simulink model "Three_point_guidance_law"  (R2024b)
settings: Solver=FixedStepAuto  StartTime=0.0  StopTime=200  FixedStep=0.01  RelTol=1e-3
settings Model: Creator=Acer  LastModifiedBy=Acer
settings DataIOCC: ReturnWorkspaceOutputs=off

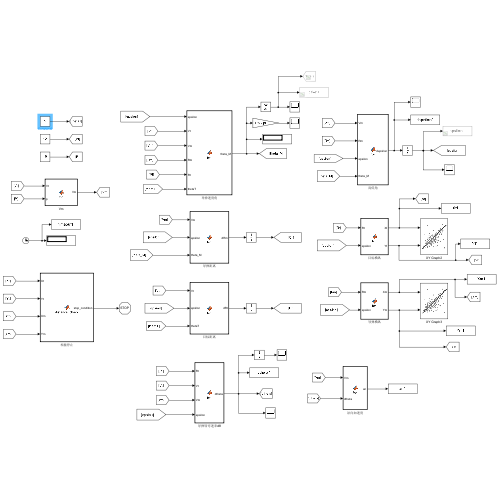
[thumbnail: Simulink's stored preview of the top-level diagram]
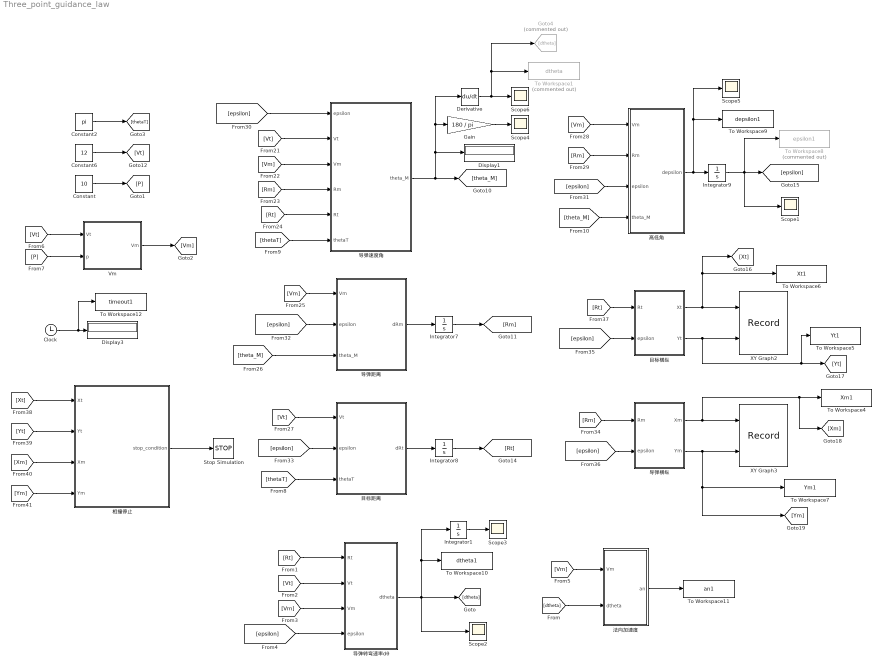
== system Three_point_guidance_law ==
  Clock : Clock
  Constant : Constant  Value=10
  Constant2 : Constant  Value=pi
  Constant6 : Constant  Value=12
  Derivative : Derivative
  Display1 : Display
  Display3 : Display
  Gain : Gain  Gain=180 / pi
  Goto4 : Goto  Commented=on  GotoTag=dtheta
  Integrator1 : Integrator  InitialCondition=70 * pi / 180
  Integrator7 : Integrator  InitialCondition=50
  Integrator8 : Integrator  InitialCondition=3000
  Integrator9 : Integrator  InitialCondition=70 * pi / 180
  Scope{1..6} (6 alike) : Scope
  Stop Simulation : Stop
  To Workspace1 : ToWorkspace  Commented=on  VariableName=dtheta  SaveFormat=Timeseries  SampleTime=-1
  To Workspace10 : ToWorkspace  VariableName=dtheta1  SaveFormat=Timeseries  SampleTime=-1
  To Workspace11 : ToWorkspace  VariableName=an1  SaveFormat=Timeseries  SampleTime=-1
  To Workspace12 : ToWorkspace  VariableName=timeout1  SaveFormat=Timeseries  SampleTime=-1
  To Workspace4 : ToWorkspace  VariableName=Xm1  SaveFormat=Timeseries  SampleTime=-1
  To Workspace5 : ToWorkspace  VariableName=Yt1  SaveFormat=Timeseries  SampleTime=-1
  To Workspace6 : ToWorkspace  VariableName=Xt1  SaveFormat=Timeseries  SampleTime=-1
  To Workspace7 : ToWorkspace  VariableName=Ym1  SaveFormat=Timeseries  SampleTime=-1
  To Workspace8 : ToWorkspace  Commented=on  VariableName=epsilon1  SaveFormat=Timeseries  SampleTime=-1
  To Workspace9 : ToWorkspace  VariableName=depsilon1  SaveFormat=Timeseries  SampleTime=-1
  Vm : MATLAB Function  TreatAsAtomicUnit=on
  XY Graph2 : Record  FileSettingsInternal="{\"entries\":[{\"content\":{\"excelSettings\":{\"content\":{},\"type\":\"Streamout.ExcelSettings\"}},\"type\":\"Streamout.FileSettingStorage\",\"uuid\":\"\"}],\"packageUris\":[\"http:\\/\\/schema.mathworks.com\\/mf0\\/streamout_blocks\\/R2020a\"],\"version\":\"1.0\"}"  Layout=[1 1]  SignalsInternal="{\"entries\":[{\"content\":{\"signals\":[{\"content\":{\"blockPath\":[],\"dimensions\":[1],\"domain\":\"\",\"lineColor\":\"#a2142f\",\"plots\":[ 1 ],\"port\":1,\"signalID\":1,\"signalName\":\"目标横纵:1\"},\"type\":\"RecordBlkView.Signal\",\"uuid\":\"\"},{\"content\":{\"blockPath\":[],\"dimensions\":[1],\"domain\":\"\",\"lineColor\":\"#139fff\",\"plots\":[ 1 ],\"port\":2,\"signalID\":2,\"signalName\":\"目标横纵:2\"},\"type\":\"RecordBlkView.Signal\",\"uuid\":\"\"}]},\"type\":\"RecordBlkView.InputSignals\",\"uuid\":\"\"}],\"packageUris\":[\"http:\\/\\/schema.mathworks.com\\/mf0\\/streamout_blocks\\/R2020a\"],\"version\":\"1.0\"}"  VisualizationBindings="{\"xyplotplugin\":{\"info\":[{\"series\":[{\"bindingParametersList\":[{\"parameter\":\"X-Axis\",\"signalID\":1,\"signalName\":\"目标横纵:1\"},{\"parameter\":\"Y-Axis\",\"signalID\":2,\"signalName\":\"目标横纵:2\"}],\"seriesID\":0}],\"subplotID\":1}]}}"  CompatibilityTag=XY
  XY Graph3 : Record  FileSettingsInternal="{\"entries\":[{\"content\":{\"excelSettings\":{\"content\":{},\"type\":\"Streamout.ExcelSettings\"}},\"type\":\"Streamout.FileSettingStorage\",\"uuid\":\"\"}],\"packageUris\":[\"http:\\/\\/schema.mathworks.com\\/mf0\\/streamout_blocks\\/R2020a\"],\"version\":\"1.0\"}"  Layout=[1 1]  SignalsInternal="{\"entries\":[{\"content\":{\"signals\":[{\"content\":{\"blockPath\":[],\"dimensions\":[1],\"domain\":\"\",\"lineColor\":\"#a2142f\",\"plots\":[ 1 ],\"port\":1,\"signalID\":1,\"signalName\":\"导弹横纵:1\"},\"type\":\"RecordBlkView.Signal\",\"uuid\":\"\"},{\"content\":{\"blockPath\":[],\"dimensions\":[1],\"domain\":\"\",\"lineColor\":\"#139fff\",\"plots\":[ 1 ],\"port\":2,\"signalID\":2,\"signalName\":\"导弹横纵:2\"},\"type\":\"RecordBlkView.Signal\",\"uuid\":\"\"}]},\"type\":\"RecordBlkView.InputSignals\",\"uuid\":\"\"}],\"packageUris\":[\"http:\\/\\/schema.mathworks.com\\/mf0\\/streamout_blocks\\/R2020a\"],\"version\":\"1.0\"}"  VisualizationBindings="{\"xyplotplugin\":{\"info\":[{\"series\":[{\"bindingParametersList\":[{\"parameter\":\"X-Axis\",\"signalID\":1,\"signalName\":\"导弹横纵:1\"},{\"parameter\":\"Y-Axis\",\"signalID\":2,\"signalName\":\"导弹横纵:2\"}],\"seriesID\":0}],\"subplotID\":1}]}}"  CompatibilityTag=XY
  导弹横纵 : MATLAB Function  TreatAsAtomicUnit=on
  导弹距离 : MATLAB Function  TreatAsAtomicUnit=on
  导弹转弯速率dθ : MATLAB Function  TreatAsAtomicUnit=on
  导弹速度角 : MATLAB Function  TreatAsAtomicUnit=on
  法向加速度 : MATLAB Function  TreatAsAtomicUnit=on
  目标横纵 : MATLAB Function  TreatAsAtomicUnit=on
  目标距离 : MATLAB Function  TreatAsAtomicUnit=on
  相撞停止 : MATLAB Function  TreatAsAtomicUnit=on
  高低角 : MATLAB Function  TreatAsAtomicUnit=on
  wires:
  [Vt] -> 导弹速度角/2(Vt)
  [Vm] -> 导弹速度角/3(Vm)
  [Rm] -> 导弹速度角/4(Rm)
  [Rt] -> 导弹速度角/5(Rt)
  [Vm] -> 导弹距离/1(Vm)
  导弹速度角/1(theta_M) -> Derivative/1, Gain/1, Display1/1, [theta_M]
  [theta_M] -> 导弹距离/3(theta_M)
  导弹距离/1(dRm) -> Integrator7/1
  Integrator7/1 -> [Rm]
  [Vt] -> 目标距离/1(Vt)
  Constant6/1 -> [Vt]
  Integrator8/1 -> [Rt]
  目标距离/1(dRt) -> Integrator8/1
  [Vm] -> 高低角/1(Vm)
  [Rm] -> 高低角/2(Rm)
  高低角/1(depsilon) -> Scope5/1, To Workspace9/1, Integrator9/1
  Integrator9/1 -> Scope1/1, To Workspace8/1, [epsilon]
  [epsilon] -> 导弹速度角/1(epsilon)
  [epsilon] -> 高低角/3(epsilon)
  [epsilon] -> 导弹距离/2(epsilon)
  [epsilon] -> 目标距离/2(epsilon)
  [Rm] -> 导弹横纵/1(Rm)
  [epsilon] -> 目标横纵/2(epsilon)
  [epsilon] -> 导弹横纵/2(epsilon)
  [Rt] -> 目标横纵/1(Rt)
  目标横纵/1(Xt) -> XY Graph2/1, To Workspace6/1, [Xt]
  目标横纵/2(Yt) -> To Workspace5/1, [Yt], XY Graph2/2
  导弹横纵/1(Xm) -> [Xm], To Workspace4/1, XY Graph3/1
  导弹横纵/2(Ym) -> [Ym], To Workspace7/1, XY Graph3/2
  相撞停止/1(stop_condition) -> Stop Simulation/1
  [Xt] -> 相撞停止/1(Xt)
  [Yt] -> 相撞停止/2(Yt)
  [Xm] -> 相撞停止/3(Xm)
  [Ym] -> 相撞停止/4(Ym)
  导弹转弯速率dθ/1(dtheta) -> Integrator1/1, To Workspace10/1, [dtheta], Scope2/1
  [Vm] -> 法向加速度/1(Vm)
  [dtheta] -> 法向加速度/2(dtheta)
  法向加速度/1(an) -> To Workspace11/1
  Integrator1/1 -> Scope3/1
  Clock/1 -> To Workspace12/1, Display3/1
  Constant/1 -> [P]
  [Vt] -> Vm/1(Vt)
  [P] -> Vm/2(p)
  Vm/1(Vm) -> [Vm]
  Constant2/1 -> [thetaT]
  Gain/1 -> Scope4/1
  [thetaT] -> 目标距离/3(thetaT)
  [thetaT] -> 导弹速度角/6(thetaT)
  [Rt] -> 导弹转弯速率dθ/1(Rt)
  [Vt] -> 导弹转弯速率dθ/2(Vt)
  [Vm] -> 导弹转弯速率dθ/3(Vm)
  [epsilon] -> 导弹转弯速率dθ/4(epsilon)
  Derivative/1 -> Goto4/1, To Workspace1/1, Scope6/1
  [theta_M] -> 高低角/4(theta_M)

== matlab function Three_point_guidance_law/法向加速度 ==
  data: Vm input; an output; dtheta input
function an = fcn(Vm, dtheta)
    an = Vm * dtheta;
end

== matlab function Three_point_guidance_law/导弹转弯速率dθ ==
  data: Rt input; Vt input; dtheta output; Vm input; epsilon input
function dtheta = fcn(Rt, Vt, Vm, epsilon)
    p = Vm / Vt;    
    H = Rt * sin(epsilon);
    dtheta = (2 * Vt * ((sin(epsilon))^2) / H) * (1 + cos(epsilon) / sqrt(p^2 - ((sin(epsilon))^2)));
end

== matlab function Three_point_guidance_law/Vm ==
  data: Vt input; Vm output; p input
function Vm = fcn(Vt, p)

Vm = Vt * p;

== matlab function Three_point_guidance_law/导弹速度角 ==
  data: epsilon input; theta_M output; Vt input; Vm input; Rm input; Rt input; thetaT input
function theta_M = fcn(epsilon, Vt, Vm, Rm, Rt, thetaT)

theta_M = epsilon + asin((Vt/Vm) * (Rm/Rt) * (-sin(epsilon - thetaT)));

== matlab function Three_point_guidance_law/导弹距离 ==
  data: Vm input; dRm output; epsilon input; theta_M input
function dRm = fcn(Vm, epsilon, theta_M)

dRm = Vm * cos(epsilon - theta_M);

== matlab function Three_point_guidance_law/目标距离 ==
  data: Vt input; dRt output; epsilon input; thetaT input
function dRt = fcn(Vt, epsilon, thetaT)
    dRt = Vt * cos(epsilon - thetaT);
end

== matlab function Three_point_guidance_law/高低角 ==
  data: Vm input; depsilon output; Rm input; epsilon input; theta_M input
function depsilon = fcn(Vm, Rm, epsilon, theta_M)

depsilon = -(Vm / Rm) * sin(epsilon - theta_M);

== matlab function Three_point_guidance_law/目标横纵 ==
  data: Rt input; Xt output; epsilon input; Yt output
function [Xt, Yt] = fcn(Rt, epsilon)

Xt = Rt * cos(epsilon);
Yt = Rt * sin(epsilon);

== matlab function Three_point_guidance_law/导弹横纵 ==
  data: Rm input; Xm output; epsilon input; Ym output
function [Xm, Ym] = fcn(Rm, epsilon)

Xm = Rm * cos(epsilon);
Ym = Rm * sin(epsilon);

== matlab function Three_point_guidance_law/相撞停止 ==
  data: Xt input; stop_condition output; Yt input; Xm input; Ym input
function stop_condition = distance_check(Xt, Yt, Xm, Ym)
    
    distance = sqrt((Xt - Xm)^2 + (Yt - Ym)^2);
    stop_condition = distance < 1;
    
end
